simulink model "P4_Modelo_Matricial_Coche_Pendulo"  (R2021a)
settings: Solver=ode4  StartTime=0.0  StopTime=10.0  FixedStep=1e-3  RelTol=1e-3
settings Model: Creator=diego  LastModifiedBy=diego
settings SolverCC: AlgebraicLoopSolver=TrustRegion
settings DataIOCC: ReturnWorkspaceOutputs=off
settings DebuggingCC: SFMachineParentedDataDiag=warning  UnderSpecifiedDimensionMsg=warning  ArithmeticOperatorsInVariantConditions=warning
settings SFSimCC: CustomCodeUndefinedFunction=UseInterfaceOnly

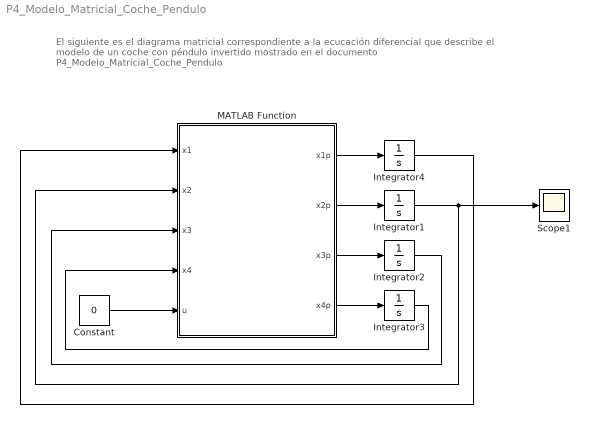
== system P4_Modelo_Matricial_Coche_Pendulo ==
  note: El siguiente es el diagrama matricial correspondiente a la ecucación diferencial que describe el modelo de un coche con péndulo invertido mostrado en el documento P4_Modelo_Matricial_Coche_Pendulo
  Constant : Constant  Value=0
  Integrator1 : Integrator  InitialCondition=pi-0.01
  Integrator2 : Integrator
  Integrator3 : Integrator
  Integrator4 : Integrator
  MATLAB Function : MATLAB Function  TreatAsAtomicUnit=on
  Scope1 : Scope
  wires:
  Constant/1 -> MATLAB Function/5(u)
  MATLAB Function/2(x2p) -> Integrator1/1
  MATLAB Function/3(x3p) -> Integrator2/1
  MATLAB Function/4(x4p) -> Integrator3/1
  Integrator3/1 -> MATLAB Function/4(x4)
  Integrator2/1 -> MATLAB Function/3(x3)
  Integrator1/1 -> Scope1/1, MATLAB Function/2(x2)
  MATLAB Function/1(x1p) -> Integrator4/1
  Integrator4/1 -> MATLAB Function/1(x1)

== matlab function P4_Modelo_Matricial_Coche_Pendulo/MATLAB Function ==
  data: x1 input; x1p output; x2 input; x3 input; x4 input; x2p output; x3p output; x4p output; u input
function [x1p,x2p,x3p,x4p] = fcn(x1,x2,x3,x4,u)
l=0.3;%Longitud péndulo [metros]
m2=0.3;%Masa del péndulo [kg]
m1=0.3;%Masa del carro [kg]
b1=0.01;%Constante de amortiguamiento de la fricción del carro
b2=0.01;%Constante de amortiguamiento de la fricción del pendulo
g=9.81;%gravedad

x1p=x3;
x2p=x4;
x3p=(l*u + b2*x4*cos(x2) - b1*l*x3 + l^2*m2*x4^2*sin(x2) - g*l*m2*cos(x2)*sin(x2))/(l*(m1 + m2) - l*m2*cos(x2)^2);
x4p=(b2*x4*(m1 + m2) + l*m2*u*cos(x2) + l^2*m2^2*x4^2*cos(x2)*sin(x2) - g*l*m2*sin(x2)*(m1 + m2) - b1*l*m2*x3*cos(x2))/(l^2*m2^2*cos(x2)^2 - l^2*m2*(m1 + m2));
end
